simulink library "randcodes"  (Simulink 5.0)
libraries: commseqgen2 x4, randcodes x1
settings Model: Creator=akansal  LastModifiedBy=akansal  ProdHWCharacteristics=Microprocessor

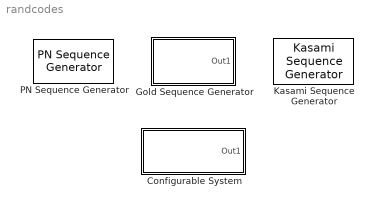
== system randcodes ==
  Configurable System : Subsystem  BlockChoice=Gold Sequence Generator
      settings: TemplateBlock=self  MemberBlocks=Gold Sequence Generator,Kasami Sequence Generator,PN Sequence Generator
  Gold Sequence Generator : Subsystem  AncestorBlock=commseqgen2/Gold Sequence Generator  mask(Gold Sequence Generator){genPoly1=[1 0 0 0 0 1 1], iniState1=[0 0 0 0 0 1], genPoly2=[1 1 0 0 1 1 1], iniState2=[0 0 0 0 0 1], index=0, shift=0, ts=1, frameBased=off, sampPerFrame=1, reset=off}
      mask prompts: genPoly1 "Preferred polynomial (1):"; iniState1 "Initial states (1):"; genPoly2 "Preferred polynomial (2):"; iniState2 "Initial states (2):"; index "Sequence index:"; ts "Sample time:"; frameBased "Frame-based outputs"; sampPerFrame "Samples per frame:"; reset "Reset on nonzero input"
      mask help:
      | Generate a Gold sequence from a set of sequences by specifying a preferred pair of polynomials.
      |
      |
      | The polynomial parameter values represent the shift register connections. Enter these values as either a binary vector or a descending ordered polynomial to indicate the connection points.
      |
      |
      | The initial states parameters are binary vectors that represent the starting state of the shift registers.
      |
      |
      | The sequence index parameter denotes the single sequence outputted from the set of Gold sequences. Specify it as a scalar integer in the range [-2, 2^n-2] where n is the degree of the generator polynomial. The index values -2 and -1 correspond to the first and second PN sequences as generated by the preferred polynomials (1) and (2), respectively.
      |
      |
      | The shift parameter is a scalar integer that produces an offset in the sequence.
      mask init:
      | [genPoly1, iniState1, genPoly2, iniState2, index, shift, rstPortLbl, eStr] = commblkgcgen(gcb, 'init');
      | 
      | if (eStr.ecode == 1)
      | 
      | 	error(eStr.emsg);
      | 
      | end
      mask Help: helpview(commbhelp);
      mask CallbackString: |||||||commblkgcgen(gcb,'cbFrameBased');||commblkgcgen(gcb,'cbReset');
      mask Display:
      | disp('Gold Sequence\nGenerator');
      | 
      | text(0.03, 0.5, rstPortLbl);
  Kasami Sequence Generator : commseqgen2/Kasami Sequence Generator  genPoly=[1 0 0 0 0 1 1]  iniState=[0 0 0 0 0 1]  codeIdx=0  shift=0  ts=1  frameBased=off  sampPerFrame=1  reset=off
  PN Sequence Generator : commseqgen2/PN Sequence Generator  poly=[1 0 0 0 0 1 1]  ini_sta=[0 0 0 0 0 1]  shift=0  Ts=1  frameBased=off  sampPerFrame=1  reset=off

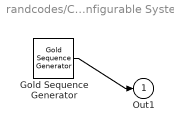
== system randcodes/Configurable System ==
  Gold Sequence Generator : randcodes/Gold Sequence Generator  AncestorBlock=commseqgen2/Gold Sequence Generator  genPoly1=[1 0 0 0 0 1 1]  iniState1=[0 0 0 0 0 1]  genPoly2=[1 1 0 0 1 1 1]  iniState2=[0 0 0 0 0 1]  index=0  shift=0  ts=1  frameBased=off  sampPerFrame=1  reset=off
  Out1 : Outport
  wires:
  Gold Sequence Generator/1 -> Out1/1

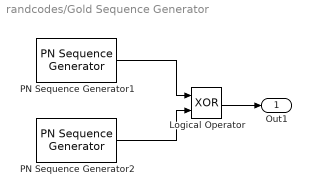
== system randcodes/Gold Sequence Generator ==
  Logical Operator : Logic  Operator=XOR  ShowAdditionalParam=on  OutDataTypeMode=Specify via dialog  LogicDataType=float('double')
  PN Sequence Generator1 : commseqgen2/PN Sequence Generator  poly=genPoly1  ini_sta=iniState1  shift=shift  Ts=ts  frameBased=off  sampPerFrame=sampPerFrame  reset=off
  PN Sequence Generator2 : commseqgen2/PN Sequence Generator  poly=genPoly2  ini_sta=iniState2  shift=shift + index  Ts=ts  frameBased=off  sampPerFrame=sampPerFrame  reset=off
  Out1 : Outport
  wires:
  Logical Operator/1 -> Out1/1
  PN Sequence Generator2/1 -> Logical Operator/2
  PN Sequence Generator1/1 -> Logical Operator/1
